simulink model "g24_5lcsc_fcsmpc"  (R2026a)
settings: Solver=VariableStepAuto  StopTime=0.08
libraries: fl_lib x26, nesl_utility x19
settings Model: Creator=yuzhuoli  LastModifiedBy=yuzhuoli

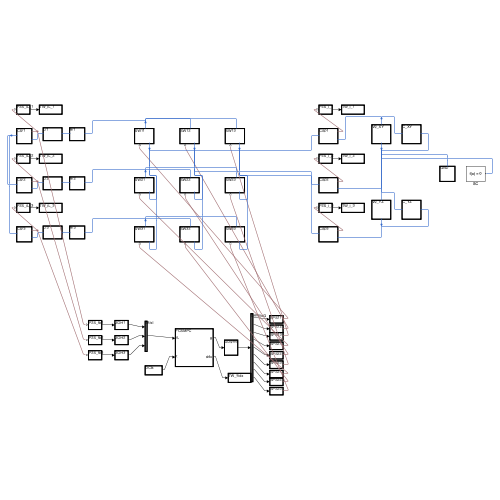
[thumbnail: Simulink's stored preview of the top-level diagram]
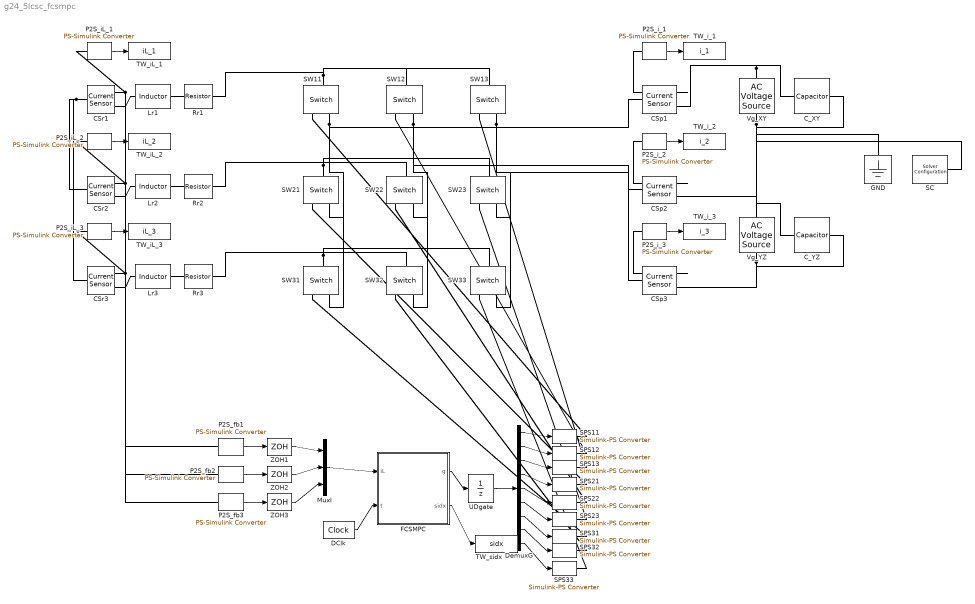
== system g24_5lcsc_fcsmpc ==
  CSp1 : fl_lib/Electrical/Electrical Sensors/Current Sensor
  CSp2 : fl_lib/Electrical/Electrical Sensors/Current Sensor
  CSp3 : fl_lib/Electrical/Electrical Sensors/Current Sensor
  CSr1 : fl_lib/Electrical/Electrical Sensors/Current Sensor
  CSr2 : fl_lib/Electrical/Electrical Sensors/Current Sensor
  CSr3 : fl_lib/Electrical/Electrical Sensors/Current Sensor
  C_XY : fl_lib/Electrical/Electrical Elements/Capacitor  c=1e-05 F  r=1e-6 Ohm  g=0 1/Ohm  i_specify=off  i_priority=None  i=0 A  i_nominal_specify=off  i_nominal_value=1  i_nominal_unit=A  v_specify=off  v_priority=None  v=0 V  v_nominal_specify=off  v_nominal_value=1  v_nominal_unit=V  vc_specify=off  vc_priority=High  vc=0 V  vc_nominal_specify=off  vc_nominal_value=1  vc_nominal_unit=V
  C_YZ : fl_lib/Electrical/Electrical Elements/Capacitor  c=1e-05 F  r=1e-6 Ohm  g=0 1/Ohm  i_specify=off  i_priority=None  i=0 A  i_nominal_specify=off  i_nominal_value=1  i_nominal_unit=A  v_specify=off  v_priority=None  v=0 V  v_nominal_specify=off  v_nominal_value=1  v_nominal_unit=V  vc_specify=off  vc_priority=High  vc=0 V  vc_nominal_specify=off  vc_nominal_value=1  vc_nominal_unit=V
  DClk : DigitalClock  SampleTime=2e-05
  DemuxG : Demux  Outputs=9
  FCSMPC : MATLAB Function  TreatAsAtomicUnit=on
  GND : fl_lib/Electrical/Electrical Elements/Electrical Reference
  Lr1 : fl_lib/Electrical/Electrical Elements/Inductor  l=0.005 H  r=0 Ohm  g=1e-9 1/Ohm  i_specify=off  i_priority=None  i=0 A  i_nominal_specify=off  i_nominal_value=1  i_nominal_unit=A  v_specify=off  v_priority=None  v=0 V  v_nominal_specify=off  v_nominal_value=1  v_nominal_unit=V  i_L_specify=off  i_L_priority=High  i_L=0 A  i_L_nominal_specify=off  i_L_nominal_value=1  i_L_nominal_unit=A
  Lr2 : fl_lib/Electrical/Electrical Elements/Inductor  l=0.005 H  r=0 Ohm  g=1e-9 1/Ohm  i_specify=off  i_priority=None  i=0 A  i_nominal_specify=off  i_nominal_value=1  i_nominal_unit=A  v_specify=off  v_priority=None  v=0 V  v_nominal_specify=off  v_nominal_value=1  v_nominal_unit=V  i_L_specify=off  i_L_priority=High  i_L=0 A  i_L_nominal_specify=off  i_L_nominal_value=1  i_L_nominal_unit=A
  Lr3 : fl_lib/Electrical/Electrical Elements/Inductor  l=0.005 H  r=0 Ohm  g=1e-9 1/Ohm  i_specify=off  i_priority=None  i=0 A  i_nominal_specify=off  i_nominal_value=1  i_nominal_unit=A  v_specify=off  v_priority=None  v=0 V  v_nominal_specify=off  v_nominal_value=1  v_nominal_unit=V  i_L_specify=off  i_L_priority=High  i_L=0 A  i_L_nominal_specify=off  i_L_nominal_value=1  i_L_nominal_unit=A
  MuxI : Mux  Inputs=3
  P2S_fb1 : nesl_utility/PS-Simulink Converter  PhysicalDomain=network_engine_domain  SubClassName=ps_output  LeftPortType=input  RightPortType=output  PseudoPeriodic=off  Frequencies=[]  VectorFormat=inherit  Unit=inherit  AffineConversion=off
  P2S_fb2 : nesl_utility/PS-Simulink Converter  PhysicalDomain=network_engine_domain  SubClassName=ps_output  LeftPortType=input  RightPortType=output  PseudoPeriodic=off  Frequencies=[]  VectorFormat=inherit  Unit=inherit  AffineConversion=off
  P2S_fb3 : nesl_utility/PS-Simulink Converter  PhysicalDomain=network_engine_domain  SubClassName=ps_output  LeftPortType=input  RightPortType=output  PseudoPeriodic=off  Frequencies=[]  VectorFormat=inherit  Unit=inherit  AffineConversion=off
  P2S_iL_1 : nesl_utility/PS-Simulink Converter  PhysicalDomain=network_engine_domain  SubClassName=ps_output  LeftPortType=input  RightPortType=output  PseudoPeriodic=off  Frequencies=[]  VectorFormat=inherit  Unit=inherit  AffineConversion=off
  P2S_iL_2 : nesl_utility/PS-Simulink Converter  PhysicalDomain=network_engine_domain  SubClassName=ps_output  LeftPortType=input  RightPortType=output  PseudoPeriodic=off  Frequencies=[]  VectorFormat=inherit  Unit=inherit  AffineConversion=off
  P2S_iL_3 : nesl_utility/PS-Simulink Converter  PhysicalDomain=network_engine_domain  SubClassName=ps_output  LeftPortType=input  RightPortType=output  PseudoPeriodic=off  Frequencies=[]  VectorFormat=inherit  Unit=inherit  AffineConversion=off
  P2S_i_1 : nesl_utility/PS-Simulink Converter  PhysicalDomain=network_engine_domain  SubClassName=ps_output  LeftPortType=input  RightPortType=output  PseudoPeriodic=off  Frequencies=[]  VectorFormat=inherit  Unit=inherit  AffineConversion=off
  P2S_i_2 : nesl_utility/PS-Simulink Converter  PhysicalDomain=network_engine_domain  SubClassName=ps_output  LeftPortType=input  RightPortType=output  PseudoPeriodic=off  Frequencies=[]  VectorFormat=inherit  Unit=inherit  AffineConversion=off
  P2S_i_3 : nesl_utility/PS-Simulink Converter  PhysicalDomain=network_engine_domain  SubClassName=ps_output  LeftPortType=input  RightPortType=output  PseudoPeriodic=off  Frequencies=[]  VectorFormat=inherit  Unit=inherit  AffineConversion=off
  Rr1 : fl_lib/Electrical/Electrical Elements/Resistor  R=0.05 Ohm  i_specify=off  i_priority=None  i=0 A  i_nominal_specify=off  i_nominal_value=1  i_nominal_unit=A  v_specify=off  v_priority=None  v=0 V  v_nominal_specify=off  v_nominal_value=1  v_nominal_unit=V
  Rr2 : fl_lib/Electrical/Electrical Elements/Resistor  R=0.05 Ohm  i_specify=off  i_priority=None  i=0 A  i_nominal_specify=off  i_nominal_value=1  i_nominal_unit=A  v_specify=off  v_priority=None  v=0 V  v_nominal_specify=off  v_nominal_value=1  v_nominal_unit=V
  Rr3 : fl_lib/Electrical/Electrical Elements/Resistor  R=0.05 Ohm  i_specify=off  i_priority=None  i=0 A  i_nominal_specify=off  i_nominal_value=1  i_nominal_unit=A  v_specify=off  v_priority=None  v=0 V  v_nominal_specify=off  v_nominal_value=1  v_nominal_unit=V
  SC : nesl_utility/Solver Configuration  PhysicalDomain=network_engine_domain  SubClassName=solver  LeftPortType=input  RightPortType=generic  Tones=[]  Harmonics=[]  SimulateNoise=off  Profile=off  UseLocalSampling=off  EnableSwitchedLinearOptims=on  FrequencyDomain=off  UseCCode=off  RelTol=0.001  AbsTol=0.001  MinStep=1e-09  ToWorkspace=off  RevertToSquareIcSolve=off  NumHomotopyIterations=100  PhasorMode=off  PhasorModeNumHarmonics=1  ConsistencySolver=NEWTON_XTOL_AFTER_FTOL  CanonicalOrdering=CANONICAL  OptimizeIntermediates=OPTIMIZED  IndexReductionMethod=DerivativeReplacement  DoDC=off  ResidualTolerance=1e-09  ConsistencyTolSource=GLOBAL  ConsistencyAbsTol=0.001  ConsistencyRelTol=0.001  ConsistencyTolFactor=0.001  UseLocalSolver=off  LocalSolverChoice=NE_BACKWARD_EULER_ADVANCER  ResolveIndetEquations=on  FunctionEvalNumThread=1  LocalSolverSampleTime=0.001  DoFixedCost=off  MaxNonlinIter=3  MaxModeIter=2  ComputeImpulses=off  ImpulseIterations=2  LinearAlgebra=auto  LinearAlgebraNumThread=0  EquationFormulation=NE_TIME_EF  DelaysMemoryBudget=1024  AutomaticFiltering=on  FilteringTimeConstant=0.001  PartitionStorageMethod=AS_NEEDED  PartitionMemoryBudget=1024  PartitionMethod=ROBUST  MultibodyUseLocalSolver=off  MultibodyLocalSolverChoice=ODE1  MultibodyLocalSolverSampleTime=0.001
  SPS{11..13,21..23,31..33} (9 alike) : nesl_utility/Simulink-PS Converter  PhysicalDomain=network_engine_domain  SubClassName=ps_input  LeftPortType=input  RightPortType=output  PseudoPeriodic=off  Frequencies=[]  NoiseDistribution=none  NoiseParameters=[]  Unit=1  AffineConversion=off  FilteringAndDerivatives=zero  SimscapeFilterOrder=1  InputFilterTimeConstant=0.001  UdotUserProvided=0
  SW{11..13,21..23,31..33} (9 alike) : fl_lib/Electrical/Electrical Elements/Switch  R_closed=0.0001 Ohm  G_open=1e-8 1/Ohm  Threshold=0.5  i_specify=off  i_priority=None  i=0 A  i_nominal_specify=off  i_nominal_value=1  i_nominal_unit=A  v_specify=off  v_priority=None  v=0 V  v_nominal_specify=off  v_nominal_value=1  v_nominal_unit=V
  TW_iL_1 : ToWorkspace  VariableName=iL_1  SampleTime=[1e-6 5e-7]
  TW_iL_2 : ToWorkspace  VariableName=iL_2  SampleTime=[1e-6 5e-7]
  TW_iL_3 : ToWorkspace  VariableName=iL_3  SampleTime=[1e-6 5e-7]
  TW_i_1 : ToWorkspace  VariableName=i_1  SampleTime=[1e-6 5e-7]
  TW_i_2 : ToWorkspace  VariableName=i_2  SampleTime=[1e-6 5e-7]
  TW_i_3 : ToWorkspace  VariableName=i_3  SampleTime=[1e-6 5e-7]
  TW_sidx : ToWorkspace  VariableName=sidx  SampleTime=2e-05
  UDgate : UnitDelay  InitialCondition=[0;1;0;0;1;0;0;1;0]  SampleTime=2e-05
  Vg_XY : fl_lib/Electrical/Electrical Sources/AC Voltage Source  amp=207.8461 V  shift=30 deg  frequency=50 Hz
  Vg_YZ : fl_lib/Electrical/Electrical Sources/AC Voltage Source  amp=207.8461 V  shift=-90 deg  frequency=50 Hz
  ZOH1 : ZeroOrderHold  SampleTime=2e-05
  ZOH2 : ZeroOrderHold  SampleTime=2e-05
  ZOH3 : ZeroOrderHold  SampleTime=2e-05
  wires:
  P2S_iL_1/1 -> TW_iL_1/1
  P2S_iL_2/1 -> TW_iL_2/1
  P2S_iL_3/1 -> TW_iL_3/1
  P2S_i_1/1 -> TW_i_1/1
  P2S_i_2/1 -> TW_i_2/1
  P2S_i_3/1 -> TW_i_3/1
  P2S_fb1/1 -> ZOH1/1
  ZOH1/1 -> MuxI/1
  P2S_fb2/1 -> ZOH2/1
  ZOH2/1 -> MuxI/2
  P2S_fb3/1 -> ZOH3/1
  ZOH3/1 -> MuxI/3
  MuxI/1 -> FCSMPC/1(iL)
  DClk/1 -> FCSMPC/2(t)
  FCSMPC/1(g) -> UDgate/1
  UDgate/1 -> DemuxG/1
  DemuxG/1 -> SPS11/1
  DemuxG/2 -> SPS12/1
  DemuxG/3 -> SPS13/1
  DemuxG/4 -> SPS21/1
  DemuxG/5 -> SPS22/1
  DemuxG/6 -> SPS23/1
  DemuxG/7 -> SPS31/1
  DemuxG/8 -> SPS32/1
  DemuxG/9 -> SPS33/1
  FCSMPC/2(sidx) -> TW_sidx/1
  connections:
  CSr1/RConn2 -- Lr1/LConn1
  Lr1/RConn1 -- Rr1/LConn1
  P2S_iL_1/LConn1 -- CSr1/RConn1 -- P2S_fb1/LConn1
  CSr2/RConn2 -- Lr2/LConn1
  Lr2/RConn1 -- Rr2/LConn1
  P2S_iL_2/LConn1 -- CSr2/RConn1 -- P2S_fb2/LConn1
  CSr3/RConn2 -- Lr3/LConn1
  Lr3/RConn1 -- Rr3/LConn1
  P2S_iL_3/LConn1 -- CSr3/RConn1 -- P2S_fb3/LConn1
  CSp1/RConn1 -- P2S_i_1/LConn1
  CSp2/RConn1 -- P2S_i_2/LConn1
  CSp3/RConn1 -- P2S_i_3/LConn1
  SPS11/RConn1 -- SW11/RConn1
  SPS12/RConn1 -- SW12/RConn1
  SPS13/RConn1 -- SW13/RConn1
  SPS21/RConn1 -- SW21/RConn1
  SPS22/RConn1 -- SW22/RConn1
  SPS23/RConn1 -- SW23/RConn1
  SPS31/RConn1 -- SW31/RConn1
  SPS32/RConn1 -- SW32/RConn1
  SPS33/RConn1 -- SW33/RConn1
  CSr2/LConn1 -- CSr1/LConn1 -- CSr3/LConn1
  C_XY/LConn1 -- Vg_XY/LConn1 -- CSp1/RConn2
  Vg_YZ/LConn1 -- Vg_XY/RConn1 -- C_XY/RConn1 -- C_YZ/LConn1 -- CSp2/RConn2 -- GND/LConn1 -- SC/RConn1
  C_YZ/RConn1 -- Vg_YZ/RConn1 -- CSp3/RConn2
  SW21/RConn2 -- SW11/RConn2 -- SW31/RConn2 -- CSp1/LConn1
  SW22/RConn2 -- SW12/RConn2 -- SW32/RConn2 -- CSp2/LConn1
  SW23/RConn2 -- SW13/RConn2 -- SW33/RConn2 -- CSp3/LConn1
  SW12/LConn1 -- SW11/LConn1 -- SW13/LConn1 -- Rr1/RConn1
  SW22/LConn1 -- SW21/LConn1 -- SW23/LConn1 -- Rr2/RConn1
  SW32/LConn1 -- SW31/LConn1 -- SW33/LConn1 -- Rr3/RConn1

== matlab function g24_5lcsc_fcsmpc/FCSMPC ==
  data: iL input; g output; t input; sidx output
function [g, sidx] = fcsmpc(iL, t)
persistent s_prev
if isempty(s_prev), s_prev = 13; end
Vg = 120; L = 0.0050000000000000001; Rr = 0.050000000000000003; Ts = 2.0000000000000002e-05; w = 2*pi*50;
t1 = 40; t2 = 40; t3 = -80;
Iq = 72; kpE = 500; Imax = 78; Idc = 80;
wbase = 100; kb = 0; wmin = 100; wmax = 100;
i1 = iL(1); i2 = iL(2); i3 = iL(3);
% white-box adaptive balancing weight: strong only when imbalance is large
imbal = abs(i1 - i2);
wbal = wbase*(1 + kb*imbal/(Idc/40));
if wbal < wmin, wbal = wmin; end
if wbal > wmax, wbal = wmax; end
[u1,u2,u3] = vrail(s_prev, Vg, w, t);
h1 = i1 + (Ts/L)*(u1 - Rr*i1);
h2 = i2 + (Ts/L)*(u2 - Rr*i2);
h3 = i3 + (Ts/L)*(u3 - Rr*i3);
tn = t + Ts;
boot = (t < 0.03);
Estar = 0.5*L*(t1^2 + t2^2 + t3^2);
E = 0.5*L*(h1^2 + h2^2 + h3^2);
Pcmd = kpE*(Estar - E) + Rr*(h1^2 + h2^2 + h3^2);
Iact = 2*Pcmd/(3*Vg);
if Iact > Imax, Iact = Imax; elseif Iact < -Imax, Iact = -Imax; end
ir = zeros(3,1);
for p = 1:3
  th = w*tn - (p-1)*2*pi/3;
  ir(p) = -Iact*sin(th) + Iq*cos(th);
end
best = inf; sbest = 0;
for s = 0:26
  [v1,v2,v3] = vrail(s, Vg, w, tn);
  q1 = h1 + (Ts/L)*(v1 - Rr*h1);
  q2 = h2 + (Ts/L)*(v2 - Rr*h2);
  q3 = h3 + (Ts/L)*(v3 - Rr*h3);
  if boot
    J = (q1-t1)^2 + (q2-t2)^2 + (q3-t3)^2;
  else
    pa = floor(s/9); pb = mod(floor(s/3),3); pc = mod(s,3);
    j1 = 0; j2 = 0; j3 = 0;
    if pa==0, j1=j1+q1; elseif pa==1, j2=j2+q1; else, j3=j3+q1; end
    if pb==0, j1=j1+q2; elseif pb==1, j2=j2+q2; else, j3=j3+q2; end
    if pc==0, j1=j1+q3; elseif pc==1, j2=j2+q3; else, j3=j3+q3; end
    J = (j1-ir(1))^2 + (j2-ir(2))^2 + (j3-ir(3))^2 + wbal*(q1-q2)^2;
  end
  if J < best, best = J; sbest = s; end
end
pa = floor(sbest/9); pb = mod(floor(sbest/3),3); pc = mod(sbest,3);
g = zeros(9,1);
g(0*3+pa+1) = 1; g(1*3+pb+1) = 1; g(2*3+pc+1) = 1;
sidx = sbest + 1;
s_prev = sbest;
end
function [v1,v2,v3] = vrail(s, Vg, w, t)
pa = floor(s/9); pb = mod(floor(s/3),3); pc = mod(s,3);
ga = Vg*sin(w*t - pa*2*pi/3);
gb = Vg*sin(w*t - pb*2*pi/3);
gc = Vg*sin(w*t - pc*2*pi/3);
cm = (ga+gb+gc)/3;
v1 = cm-ga; v2 = cm-gb; v3 = cm-gc;
end
